simulink model "SoftStop_Standalone"  (R2022b)
settings: Solver=VariableStepAuto  StartTime=0.0  StopTime=10.0  RelTol=1e-3
undefined symbols (not defined in the file): AntiJerk_rear, iStop_Axle, iStop_ComfStop_Axis_SpeedAct_HA, iStop_ComfStop_Axis_SpeedActVA, iStop_ComfStop_TrqMinCont_HA, iStop_ComfStop_TrqMinCont_VA, iStop_HillComp_Axis_Steigung1, iStop_HillComp_Axis_Steigung2, iStop_HillComp_CompTrqFacHA, iStop_HillComp_CompTrqFacVA, iStop_HillComp_HillCompTrq, iStop_HillComp_HillEntrySpd, iStop_HillComp_HillExitPrs, iStop_HillComp_HillTrqLim_Dec_NegGrd, iStop_HillComp_HillTrqLim_Dec_PosGrd, iStop_HillComp_HillTrqLim_Inc_NegGrd, iStop_HillComp_HillTrqLim_Inc_PosGrd, iStop_Misc_SpeedLowr_Drive_Dir_HA, iStop_Misc_SpeedLowr_Drive_Dir_VA, iStop_Misc_SpeedUppr_Drive_Dir_HA, iStop_Misc_SpeedUppr_Drive_Dir_VA, iStop_PosCtrl_Activate_var_gain_HA, iStop_PosCtrl_Activate_var_gain_VA, iStop_PosCtrl_Actv_SpeedLowr_HA, iStop_PosCtrl_Actv_SpeedLowr_VA, iStop_PosCtrl_Actv_SpeedUppr_HA, iStop_PosCtrl_Actv_SpeedUppr_VA, iStop_PosCtrl_Axis_BrakeTorque_HA, iStop_PosCtrl_Axis_BrakeTorque_VA, iStop_PosCtrl_Axis_Delta_Speed_HA_Line, iStop_PosCtrl_Axis_Delta_Speed_HA_Map, iStop_PosCtrl_Axis_Delta_Speed_VA_Line, iStop_PosCtrl_Axis_Delta_Speed_VA_Map, iStop_PosCtrl_Axis_SpeedAct_VA, iStop_PosCtrl_Axis_SpeedActRear, iStop_PosCtrl_Axis_SpeedFilt_HA, iStop_PosCtrl_Axis_SpeedFilt_VA, iStop_PosCtrl_Gain_Line_HA, iStop_PosCtrl_Gain_Line_VA, iStop_PosCtrl_Gain_Map_HA, iStop_PosCtrl_Gain_Map_VA, iStop_PosCtrl_Hp_Filt_HA, iStop_PosCtrl_Hp_Filt_VA, iStop_PosCtrl_TrqOutput_PT1_HA, iStop_PosCtrl_TrqOutput_PT1_VA, iStop_SpeedLowrLim_Global_Actv, iStop_SpeedUpprLim_Global_Deactv, iStop_Standstill_Activate_hp_speed_filt_HA, iStop_Standstill_Activate_hp_speed_filt_VA, iStop_Standstill_Axis_PedalTravel, iStop_Standstill_Axis_SpeedAct_HA, iStop_Standstill_Axis_SpeedAct_VA, iStop_Standstill_delayHA, iStop_Standstill_delayVA, iStop_Standstill_Hp_Filt_HA, iStop_Standstill_Hp_Filt_VA, iStop_Standstill_MaxSpeedHA, iStop_Standstill_MaxSpeedVA, iStop_Standstill_MinSpeedHA, iStop_Standstill_MinSpeedVA ... (+2)
libraries: simulink x7, simulink_extras x6
settings Model: Creator=Z0186328  LastModifiedBy=Z0186328

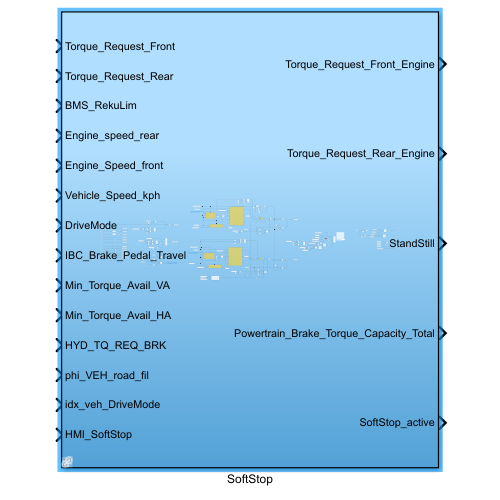
[thumbnail: Simulink's stored preview of the top-level diagram]
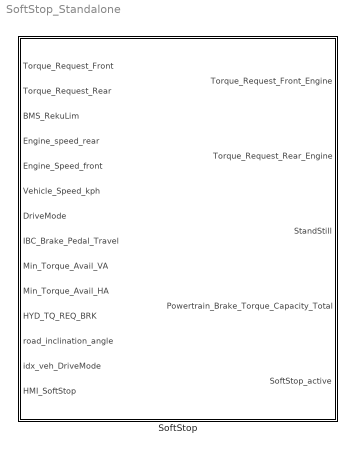
== system SoftStop_Standalone ==
  SoftStop : Subsystem  AncestorBlock=AntiJerk_rear/AntiJerk_rear

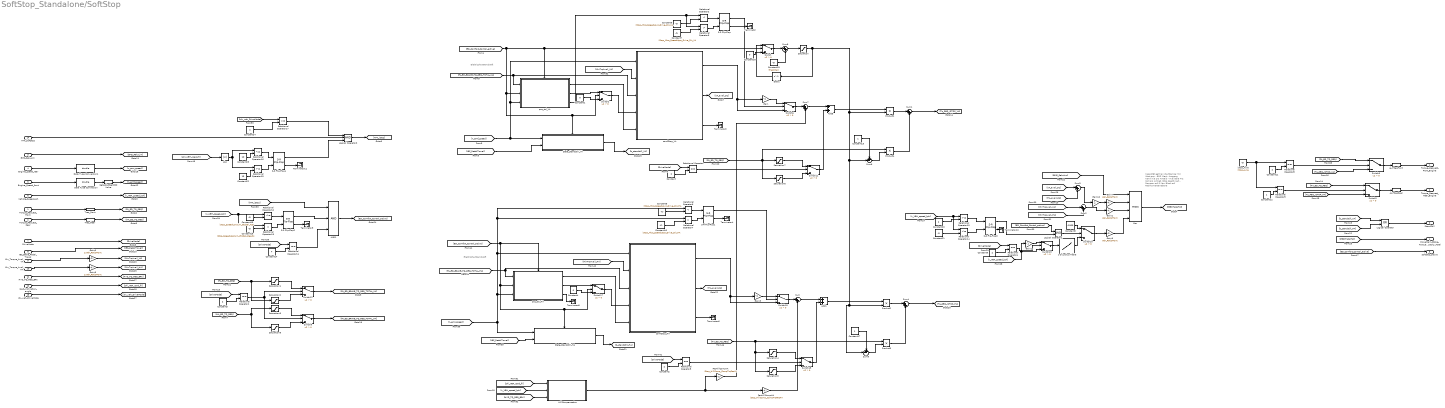
== system SoftStop_Standalone/SoftStop ==
  note: Elektrische Bremskraft
  note: Elektrische Bremskraft
  note: Kapazität geht an die Bremse:
      | Min Wert aus:
      | - BMS Wert
      | - Ausgang Kennlinie pro Antreib
      | - Available Trq CAN pro Antrieb
      |
      | IStop deaktiviert
      | - Rampen auf 0
      |
      | Max Block auf Radmomentenebene
  Torque_Request_Front : Inport
  Torque_Request_Rear : Inport  Port=2
  BMS_RekuLim : Inport  Port=3
  Engine_speed_rear : Inport  Port=4
  Engine_Speed_front : Inport  Port=5
  Vehicle_Speed_kph : Inport  Port=6
  DriveMode : Inport  Port=7
  IBC_Brake_Pedal_Travel : Inport  Port=8
  Min_Torque_Avail_VA : Inport  Port=9
  Min_Torque_Avail_HA : Inport  Port=10
  HYD_TQ_REQ_BRK : Inport  Port=11
  road_inclination_angle : Inport  Port=12
  idx_veh_DriveMode : Inport  Port=13
  HMI_SoftStop : Inport  Port=14
  1-D Lookup Table : Lookup_n-D  NumberOfTableDimensions=1  BreakpointsForDimension1=[0 8 12 15 20]  Table=[0 0 -250 -500 -1000]  ExtrapMethod=Clip  InternalRulePriority=Speed  RndMeth=Simplest
  AJ_TReqFront : SignalConversion  OverrideOpt=off
  AJ_TReqRear : SignalConversion  OverrideOpt=off
  AND1 : Logic  Inputs=3  AllPortsSameDT=off  OutDataTypeStr=boolean
  Abs : Abs  SaturateOnIntegerOverflow=off
  Add1 : Sum
  Add5 : Sum
  Constant{,2..3,9,11,20,24} (7 alike) : Constant  Value=2
  Constant1 : Constant  Value=0
  Constant10 : Constant  Value=iStop_Misc_SpeedUppr_Drive_Dir_HA
  Constant12 : Constant
  Constant13 : Constant
  Constant14 : Constant  Value=4
  Constant15 : Constant  Value=iStop_SpeedLowrLim_Global_Actv
  Constant16 : Constant  Value=iStop_SpeedUpprLim_Global_Deactv
  Constant17 : Constant
  Constant18 : Constant  Value=0
  Constant19 : Constant  Value=tTaskMain
  Constant21 : Constant  Value=-3
  Constant22 : Constant  Value=13
  Constant23 : Constant  Value=10
  Constant4 : Constant  Value=0
  Constant5 : Constant  Value=iStop_Misc_SpeedLowr_Drive_Dir_HA
  Constant6 : Constant  Value=iStop_Misc_SpeedLowr_Drive_Dir_VA
  Constant7 : Constant  Value=iStop_Misc_SpeedUppr_Drive_Dir_VA
  Constant8 : Constant  Value=-1000
  Data Type Conversion : DataTypeConversion  OutDataTypeStr=double  SaturateOnIntegerOverflow=off  RndMeth=Floor
  Data Type Conversion1 : DataTypeConversion  OutDataTypeStr=double  SaturateOnIntegerOverflow=off  RndMeth=Floor
  Delay : Delay  DelayLength=1  InitialCondition=0
  FacHillCompHA : Gain  Gain=iStop_HillComp_CompTrqFacHA
  FacHillCompVA : Gain  Gain=iStop_HillComp_CompTrqFacVA
  Gain : Gain  Gain=-1
  Gain1 : Gain  Gain=-1
  Gain10 : Gain  Gain=2
  Gain2 : Gain  Gain=Veh_RatioFront
  Gain3 : Gain  Gain=-1
  Gain6 : Gain  Gain=1/Veh_RatioFront
  Gain7 : Gain  Gain=Veh_RatioFront
  Gain8 : Gain  Gain=1/Veh_RatioFront
  Gain9 : Gain  Gain=Veh_RatioFront
  HillCompensation : Subsystem
  IsgSpdActSgn800 Value : SignalConversion  OverrideOpt=off
  Logical Operator : Logic  Operator=OR  AllPortsSameDT=off  OutDataTypeStr=boolean
  Logical Operator1 : Logic  AllPortsSameDT=off  OutDataTypeStr=boolean
  Logical Operator2 : Logic  Inputs=3  AllPortsSameDT=off  OutDataTypeStr=boolean
  Max : MinMax  Function=max  Inputs=4
  Product{1..4} (4 alike) : Product
  Relational Operator{,1,4..5,8..9,11} (7 alike) : RelationalOperator  Operator===  OutDataTypeStr=boolean  RndMeth=Simplest  InputSameDT=off
  Relational Operator10 : RelationalOperator  OutDataTypeStr=boolean  RndMeth=Simplest  InputSameDT=off
  Relational Operator{12,14,16..17} (4 alike) : RelationalOperator  Operator=<=  OutDataTypeStr=boolean  RndMeth=Simplest  InputSameDT=off
  Relational Operator13 : RelationalOperator  Operator=>  OutDataTypeStr=boolean  RndMeth=Simplest  InputSameDT=off
  Relational Operator15 : RelationalOperator  OutDataTypeStr=boolean  RndMeth=Simplest  InputSameDT=off
  Relational Operator2 : RelationalOperator  Operator=<  OutDataTypeStr=boolean  RndMeth=Simplest  InputSameDT=off
  Relational Operator3 : RelationalOperator  Operator=>  OutDataTypeStr=boolean  RndMeth=Simplest  InputSameDT=off
  Relational Operator6 : RelationalOperator  Operator=<  OutDataTypeStr=boolean  RndMeth=Simplest  InputSameDT=off
  Relational Operator7 : RelationalOperator  Operator=>  OutDataTypeStr=boolean  RndMeth=Simplest  InputSameDT=off
  S-R Flip-Flop{,1..4} (5 alike) : simulink_extras/Flip Flops/S-R Flip-Flop  initial_condition=0
  Saturation : Saturate  UpperLimit=1  LowerLimit=0
  Saturation{1,3,5..6} (4 alike) : Saturate  UpperLimit=inf  LowerLimit=0
  Saturation{2,4,7..8} (4 alike) : Saturate  UpperLimit=0  LowerLimit=-inf
  State_Standstill_HA : Subsystem
  State_Standstill_VA : Subsystem
  Sum{,1..4,7..8} (7 alike) : Sum  Inputs=|++
  Sum5 : Sum  Inputs=+-|
  Sum6 : Sum  Inputs=+-|
  Switch{,2..3,5..6,9..13,15,17..18} (13 alike) : Switch  Criteria=u2 > Threshold  SaturateOnIntegerOverflow=off  InputSameDT=off
  Terminator{,2,4,6,8..11} (8 alike) : Terminator
  Treq_Front : SignalConversion  OverrideOpt=off
  Treq_Rear : SignalConversion  OverrideOpt=off
  comfStop_HA : Subsystem
  comfStop_VA : Subsystem
  iStop_Axle : Constant  Value=iStop_Axle
  pos_ctrl_HA : Subsystem
  pos_ctrl_VA : Subsystem
  Torque_Request_Front_Engine : Outport
  Torque_Request_Rear_Engine : Outport  Port=2
  StandStill : Outport  Port=3
  Powertrain_Brake_Torque_Capacity_Total : Outport  Port=4
  SoftStop_active : Outport  Port=5
  wires:
  [ED_Comfort_Control_active] -> State_Standstill_HA/Enable, Switch17/2, pos_ctrl_HA/2(pos_ctrl_active), pos_ctrl_HA/Enable
  [ED_Comfort_Control_active] -> pos_ctrl_VA/Enable, Switch/2, Switch2/2, State_Standstill_VA/Enable, pos_ctrl_VA/2(pos_ctrl_active)
  Gain9/1 -> Max/4
  Gain7/1 -> Max/2
  Gain2/1 -> Max/3
  AJ_TReqRear/1 -> Torque_Request_Rear_Engine/1  "TReqRear"
  AJ_TReqFront/1 -> Torque_Request_Front_Engine/1  "TReqFront"
  Engine_Speed_front/1 -> Data Type Conversion/1
  Torque_Request_Rear/1 -> Treq_Rear/1
  Torque_Request_Front/1 -> Treq_Front/1
  Vehicle_Speed_kph/1 -> [v_VEH_speed_kph]
  IsgSpdActSgn800 Value/1 -> [n_emf_speed]
  Engine_speed_rear/1 -> Data Type Conversion1/1
  Saturation2/1 -> Switch12/3
  [DriveMode] -> Relational Operator1/1
  [FA_ED_TQ_REQ] -> Saturation1/1, Saturation2/1
  Saturation1/1 -> Switch12/1
  Saturation5/1 -> Switch9/1
  Saturation8/1 -> Switch9/3
  [HA_ED_TQ_REQ] -> Saturation5/1, Saturation8/1
  Relational Operator1/1 -> Switch12/2, Switch9/2
  Constant3/1 -> Relational Operator1/2
  Switch12/1 -> [FA_ED_BRAKE_TQ_REQ_TOTAL_VA]
  Switch9/1 -> [FA_ED_BRAKE_TQ_REQ_TOTAL_HA]
  [MinTrqAvail_HA] -> comfStop_HA/2(Tq_Avail_Min_HA)
  Relational Operator/1 -> Switch11/2
  Switch11/1 -> Add5/2
  Relational Operator3/1 -> S-R Flip-Flop/2
  [FA_ED_BRAKE_TQ_REQ_TOTAL_VA] -> comfStop_VA/3(ED_Brake_Tq_Req_VA_Total), pos_ctrl_VA/1(brake_torque_total)
  [DriveMode] -> Relational Operator/1
  S-R Flip-Flop/1 -> Switch6/2
  comfStop_VA/3(ED_Brake_Tq_VA_100%) -> Terminator2/1
  Constant2/1 -> Relational Operator5/2
  [DriveMode] -> Relational Operator5/1
  Constant/1 -> Relational Operator/2
  Constant6/1 -> Relational Operator2/2
  Constant7/1 -> Relational Operator3/2
  pos_ctrl_VA/3(speed_filt) -> Relational Operator2/1, Relational Operator3/1
  Relational Operator2/1 -> S-R Flip-Flop/1
  S-R Flip-Flop1/2 -> Terminator4/1
  Switch15/1 -> Add1/2
  Constant10/1 -> Relational Operator7/2
  Gain3/1 -> Switch18/1
  [n_emr_speed] -> comfStop_HA/1(Speed_Act_HA), Relational Operator7/1, Relational Operator6/1, pos_ctrl_HA/3(speed_act_HA), State_Standstill_HA/1(speed_act_HA)  "speed_act_HA"
  Relational Operator6/1 -> S-R Flip-Flop1/1
  comfStop_HA/2(HA_avail_trq) -> [HA_avail_trq]
  pos_ctrl_HA/2(position_control_trq_output_HA) -> Switch17/1
  Constant5/1 -> Relational Operator6/2
  State_Standstill_HA/1(stop_signal_after_integrator) -> [b_standstill_HA]  "stop_signal_active"
  [FA_ED_BRAKE_TQ_REQ_TOTAL_HA] -> comfStop_HA/3(ED_Brake_Tq_Req_HA_Total), pos_ctrl_HA/1(brake_torque_total)
  S-R Flip-Flop1/1 -> Switch18/2
  comfStop_HA/1(Brake_Tq_Req_HA_EDrive_Adjusted) -> Switch18/3, Gain3/1
  Saturation3/1 -> Switch15/3
  [n_emf_speed] -> State_Standstill_VA/1(speed_act_VA), pos_ctrl_VA/3(speed_act_VA), comfStop_VA/1(Speed_Act_VA)  "speed_act_VA"
  Constant4/1 -> Switch17/3
  comfStop_HA/3(ED_Brake_Tq_HA_100%) -> Terminator6/1
  [MinTrqAvail_VA] -> comfStop_VA/2(Tq_Avail_Min_VA)
  S-R Flip-Flop/2 -> Terminator/1
  Sum/1 -> Add1/1
  Gain/1 -> Switch6/1
  Saturation6/1 -> Switch11/3
  Saturation7/1 -> Switch11/1
  pos_ctrl_VA/2(position_control_trq_output_VA) -> Switch2/1
  Switch17/1 -> comfStop_HA/4(Pos_CRTL_TRQ_HA)
  Saturation4/1 -> Switch15/1
  Constant1/1 -> Switch2/3
  pos_ctrl_VA/1(pos_control_active_flag_VA) -> comfStop_VA/5(POS_CTRL_ACTIVE_VA)
  [FA_ED_TQ_REQ] -> Product4/1, Saturation6/1, Saturation7/1
  Relational Operator5/1 -> Switch15/2
  Sum7/1 -> Add5/1
  [IBC_PedalTravel] -> State_Standstill_VA/2(PedalTravel)
  Relational Operator7/1 -> S-R Flip-Flop1/2
  comfStop_VA/2(VA_avail_trq) -> [VA_avail_trq]
  pos_ctrl_HA/1(pos_control_active_flag_HA) -> comfStop_HA/5(POS_CTRL_ACTIVE_HA)
  Switch2/1 -> comfStop_VA/4(Pos_CRTL_TRQ_VA)
  comfStop_VA/1(Brake_Tq_Req_VA_EDrive_Adjusted) -> Gain/1, Switch6/3
  [IBC_PedalTravel] -> State_Standstill_HA/2(PedalTravel)
  pos_ctrl_HA/3(speed_filt) -> Terminator8/1
  State_Standstill_VA/1(stop_signal_after_integrator) -> [b_standstill_VA]  "stop_signal_active"
  1-D Lookup Table/1 -> Switch10/3
  Switch13/1 -> 1-D Lookup Table/1
  Gain1/1 -> Switch13/1
  [MinTrqAvail_VA] -> Sum2/1
  [BMS_RekuLim] -> Max/1
  Sum3/1 -> Gain10/1
  Logical Operator1/1 -> Switch10/2
  Relational Operator4/1 -> Switch13/2
  [v_VEH_speed_kph] -> Gain1/1, Switch13/3
  Constant8/1 -> Switch10/1
  Sum2/1 -> Gain2/1
  Switch10/1 -> Gain9/1
  [HA_avail_trq] -> Sum3/2
  [DriveMode] -> Relational Operator4/1
  Max/1 -> [PtBrkTqCpTot]
  Constant9/1 -> Relational Operator4/2
  [MinTrqAvail_HA] -> Sum2/2
  [VA_avail_trq] -> Sum3/1
  [b_standstill_HA] -> Logical Operator/2  "b_StandStill"
  [PtBrkTqCpTot] -> Powertrain_Brake_Torque_Capacity_Total/1  "PtBrkTqCpTot"
  [b_standstill_VA] -> Logical Operator/1  "b_StandStill"
  Switch3/1 -> AJ_TReqRear/1
  [FA_ED_TQ_REQ] -> Switch5/1
  [HA_ED_TQ_REQ] -> Switch3/1
  Switch5/1 -> AJ_TReqFront/1
  Relational Operator8/1 -> Switch5/2
  Constant12/1 -> Relational Operator9/2
  [Tq_REQ_ISTOP_HA] -> Switch3/3
  [Tq_REQ_ISTOP_VA] -> Switch5/3
  Constant11/1 -> Relational Operator8/2
  Relational Operator9/1 -> Switch3/2
  iStop_Axle/1 -> Relational Operator9/1, Relational Operator8/1
  Treq_Front/1 -> [FA_ED_TQ_REQ]  "AJ_TReqFront"
  Treq_Rear/1 -> [HA_ED_TQ_REQ]
  IBC_Brake_Pedal_Travel/1 -> [IBC_PedalTravel]
  Logical Operator2/1 -> [HMI_iStop]
  DriveMode/1 -> [DriveMode]
  BMS_RekuLim/1 -> [BMS_RekuLim]
  Min_Torque_Avail_VA/1 -> Gain6/1
  Min_Torque_Avail_HA/1 -> Gain8/1
  Gain6/1 -> [MinTrqAvail_VA]
  Gain8/1 -> [MinTrqAvail_HA]
  Logical Operator/1 -> StandStill/1  "b_StandStill"
  HYD_TQ_REQ_BRK/1 -> [HYD_TQ_REQ_BRK]  "IBC_SRBM_IST"
  Data Type Conversion1/1 -> [n_emr_speed]
  Data Type Conversion/1 -> IsgSpdActSgn800 Value/1
  Relational Operator11/1 -> AND1/3
  Constant15/1 -> Relational Operator12/2
  [v_VEH_speed_kph] -> Relational Operator12/1, Relational Operator13/1
  Constant19/1 -> Sum8/2
  Relational Operator13/1 -> S-R Flip-Flop2/2
  Switch/1 -> Sum8/1
  S-R Flip-Flop2/1 -> AND1/2
  Constant18/1 -> Switch/3
  [HMI_iStop] -> AND1/1
  Delay/1 -> Switch/1
  Sum8/1 -> Saturation/1
  AND1/1 -> [ED_Comfort_Control_active]
  [DriveMode] -> Relational Operator11/1
  Relational Operator12/1 -> S-R Flip-Flop2/1
  Constant16/1 -> Relational Operator13/2
  Constant14/1 -> Relational Operator11/2
  S-R Flip-Flop2/2 -> Terminator9/1
  Sum4/1 -> [Tq_REQ_ISTOP_HA]
  Add1/1 -> Product2/1
  Product2/1 -> Sum4/1
  Product3/1 -> Sum4/2
  [HA_ED_TQ_REQ] -> Saturation3/1, Saturation4/1, Product3/1
  Constant17/1 -> Sum5/1
  Sum5/1 -> Product3/2
  Sum6/1 -> Product4/2
  Saturation/1 -> Product1/2, Sum5/2, Product2/2, Sum6/2, Delay/1  "ED_Comfort_Control_active_interpol"
  Constant13/1 -> Sum6/1
  Product4/1 -> Sum1/2
  Product1/1 -> Sum1/1
  Add5/1 -> Product1/1
  Sum1/1 -> [Tq_REQ_ISTOP_VA]
  Switch18/1 -> Sum/1
  [v_VEH_speed_kph] -> HillCompensation/2(Speed)
  [HYD_TQ_REQ_BRK] -> HillCompensation/3(BrakePressure)
  [phi_VEH_road_fil] -> HillCompensation/1(Steigung)
  HillCompensation/1(trq_hillcomp) -> FacHillCompHA/1, FacHillCompVA/1
  road_inclination_angle/1 -> [phi_VEH_road_fil]
  [v_VEH_speed_kph] -> Relational Operator10/1, Relational Operator14/1
  S-R Flip-Flop3/2 -> Terminator10/1
  Constant21/1 -> Relational Operator14/2
  Relational Operator10/1 -> S-R Flip-Flop3/1
  [ED_Comfort_Control_active] -> Logical Operator1/1
  Relational Operator14/1 -> S-R Flip-Flop3/2
  S-R Flip-Flop3/1 -> Logical Operator1/2
  Constant20/1 -> Relational Operator10/2
  FacHillCompHA/1 -> Sum/2
  Switch6/1 -> Sum7/1
  FacHillCompVA/1 -> Sum7/2
  [ED_Comfort_Control_active] -> SoftStop_active/1  "ED_Comfort_Control_active"
  S-R Flip-Flop4/1 -> Logical Operator2/3
  S-R Flip-Flop4/2 -> Terminator11/1
  [phi_VEH_road_fil] -> Abs/1
  Relational Operator15/1 -> S-R Flip-Flop4/2
  Constant22/1 -> Relational Operator15/2
  Abs/1 -> Relational Operator16/1, Relational Operator15/1
  Relational Operator16/1 -> S-R Flip-Flop4/1
  Constant23/1 -> Relational Operator16/2
  Constant24/1 -> Relational Operator17/2
  Relational Operator17/1 -> Logical Operator2/1
  idx_veh_DriveMode/1 -> [idx_veh_DriveMode]
  [idx_veh_DriveMode] -> Relational Operator17/1
  Gain10/1 -> Gain7/1
  HMI_SoftStop/1 -> Logical Operator2/2

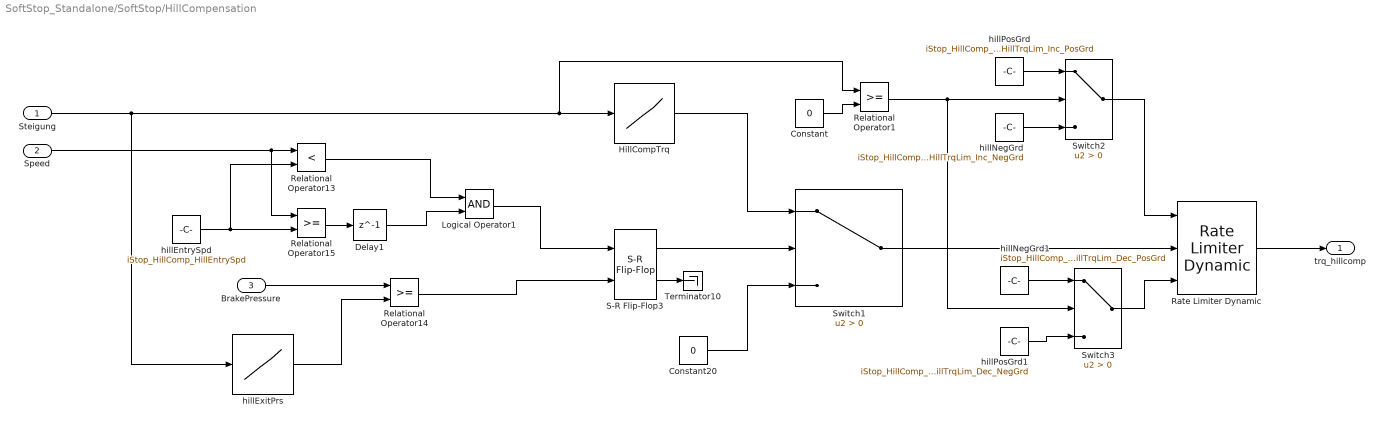
== system SoftStop_Standalone/SoftStop/HillCompensation ==
  Steigung : Inport
  Speed : Inport  Port=2
  BrakePressure : Inport  Port=3
  Constant : Constant  Value=0
  Constant20 : Constant  Value=0
  Delay1 : Delay  DelayLength=1  InitialCondition=0
  HillCompTrq : Lookup_n-D  NumberOfTableDimensions=1  BreakpointsForDimension1=iStop_HillComp_Axis_Steigung2  Table=iStop_HillComp_HillCompTrq  ExtrapMethod=Clip  UseLastTableValue=on  InternalRulePriority=Speed  RndMeth=Simplest
  Logical Operator1 : Logic  AllPortsSameDT=off  OutDataTypeStr=boolean
  Rate Limiter Dynamic : simulink/Discontinuities/Rate Limiter Dynamic
  Relational Operator1 : RelationalOperator  OutDataTypeStr=boolean  RndMeth=Simplest  InputSameDT=off
  Relational Operator13 : RelationalOperator  Operator=<  OutDataTypeStr=boolean  RndMeth=Simplest  InputSameDT=off
  Relational Operator14 : RelationalOperator  OutDataTypeStr=boolean  RndMeth=Simplest  InputSameDT=off
  Relational Operator15 : RelationalOperator  OutDataTypeStr=boolean  RndMeth=Simplest  InputSameDT=off
  S-R Flip-Flop3 : simulink_extras/Flip Flops/S-R Flip-Flop  initial_condition=0
  Switch1 : Switch  Criteria=u2 > Threshold  SaturateOnIntegerOverflow=off  InputSameDT=off
  Switch2 : Switch  Criteria=u2 > Threshold  SaturateOnIntegerOverflow=off  InputSameDT=off
  Switch3 : Switch  Criteria=u2 > Threshold  SaturateOnIntegerOverflow=off  InputSameDT=off
  Terminator10 : Terminator
  hillEntrySpd : Constant  Value=iStop_HillComp_HillEntrySpd
  hillExitPrs : Lookup_n-D  NumberOfTableDimensions=1  BreakpointsForDimension1=iStop_HillComp_Axis_Steigung1  Table=iStop_HillComp_HillExitPrs  ExtrapMethod=Clip  UseLastTableValue=on  InternalRulePriority=Speed  RndMeth=Simplest
  hillNegGrd : Constant  Value=iStop_HillComp_HillTrqLim_Inc_NegGrd
  hillNegGrd1 : Constant  Value=iStop_HillComp_HillTrqLim_Dec_PosGrd
  hillPosGrd : Constant  Value=iStop_HillComp_HillTrqLim_Inc_PosGrd
  hillPosGrd1 : Constant  Value=iStop_HillComp_HillTrqLim_Dec_NegGrd
  trq_hillcomp : Outport
  wires:
  hillPosGrd1/1 -> Switch3/3
  hillNegGrd1/1 -> Switch3/1
  Constant/1 -> Relational Operator1/2
  Relational Operator1/1 -> Switch2/2, Switch3/2
  Switch3/1 -> Rate Limiter Dynamic/3
  hillNegGrd/1 -> Switch2/3
  Switch2/1 -> Rate Limiter Dynamic/1
  hillPosGrd/1 -> Switch2/1
  BrakePressure/1 -> Relational Operator14/1
  Switch1/1 -> Rate Limiter Dynamic/2
  Logical Operator1/1 -> S-R Flip-Flop3/1
  hillExitPrs/1 -> Relational Operator14/2
  Rate Limiter Dynamic/1 -> trq_hillcomp/1
  Delay1/1 -> Logical Operator1/2
  Relational Operator14/1 -> S-R Flip-Flop3/2
  Steigung/1 -> HillCompTrq/1, Relational Operator1/1, hillExitPrs/1
  HillCompTrq/1 -> Switch1/1
  Constant20/1 -> Switch1/3
  Relational Operator15/1 -> Delay1/1
  S-R Flip-Flop3/1 -> Switch1/2
  Speed/1 -> Relational Operator13/1, Relational Operator15/1
  Relational Operator13/1 -> Logical Operator1/1
  S-R Flip-Flop3/2 -> Terminator10/1
  hillEntrySpd/1 -> Relational Operator15/2, Relational Operator13/2

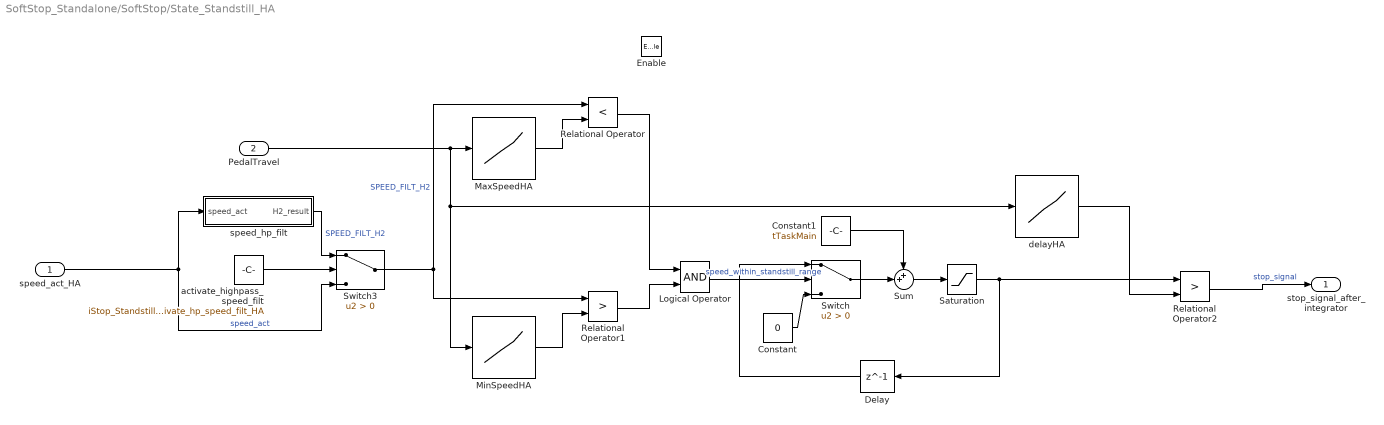
== system SoftStop_Standalone/SoftStop/State_Standstill_HA ==
  speed_act_HA : Inport
  PedalTravel : Inport  Port=2
  Enable : EnablePort  StatesWhenEnabling=reset
  Constant : Constant  Value=0
  Constant1 : Constant  Value=tTaskMain
  Delay : Delay  DelayLength=1  InitialCondition=0
  Logical Operator : Logic  AllPortsSameDT=off  OutDataTypeStr=boolean
  MaxSpeedHA : Lookup_n-D  NumberOfTableDimensions=1  BreakpointsForDimension1=iStop_Standstill_Axis_PedalTravel  Table=iStop_Standstill_MaxSpeedHA  ExtrapMethod=Clip  UseLastTableValue=on  InternalRulePriority=Speed  RndMeth=Simplest
  MinSpeedHA : Lookup_n-D  NumberOfTableDimensions=1  BreakpointsForDimension1=iStop_Standstill_Axis_PedalTravel  Table=iStop_Standstill_MinSpeedHA  ExtrapMethod=Clip  UseLastTableValue=on  InternalRulePriority=Speed  RndMeth=Simplest
  Relational Operator : RelationalOperator  Operator=<  OutDataTypeStr=boolean  RndMeth=Simplest  InputSameDT=off
  Relational Operator1 : RelationalOperator  Operator=>  OutDataTypeStr=boolean  RndMeth=Simplest  InputSameDT=off
  Relational Operator2 : RelationalOperator  Operator=>  OutDataTypeStr=boolean  RndMeth=Simplest  InputSameDT=off
  Saturation : Saturate  UpperLimit=10  LowerLimit=0
  Sum : Sum  Inputs=++|
  Switch : Switch  Criteria=u2 > Threshold  SaturateOnIntegerOverflow=off  InputSameDT=off
  Switch3 : Switch  Criteria=u2 > Threshold  SaturateOnIntegerOverflow=off  InputSameDT=off
  activate_highpass_speed_filt : Constant  Value=iStop_Standstill_Activate_hp_speed_filt_HA
  delayHA : Lookup_n-D  NumberOfTableDimensions=1  BreakpointsForDimension1=iStop_Standstill_Axis_PedalTravel  Table=iStop_Standstill_delayHA  ExtrapMethod=Clip  UseLastTableValue=on  InternalRulePriority=Speed  RndMeth=Simplest
  speed_hp_filt : Subsystem
  stop_signal_after_integrator : Outport
  wires:
  delayHA/1 -> Relational Operator2/2
  MinSpeedHA/1 -> Relational Operator1/2
  Relational Operator1/1 -> Logical Operator/2
  PedalTravel/1 -> MaxSpeedHA/1, delayHA/1, MinSpeedHA/1
  MaxSpeedHA/1 -> Relational Operator/2
  Relational Operator2/1 -> stop_signal_after_integrator/1  "stop_signal"
  Logical Operator/1 -> Switch/2  "speed_within_standstill_range"
  Relational Operator/1 -> Logical Operator/1
  speed_act_HA/1 -> Switch3/3, speed_hp_filt/1(speed_act)  "speed_act"
  speed_hp_filt/1(H2_result) -> Switch3/1  "SPEED_FILT_H2"
  activate_highpass_speed_filt/1 -> Switch3/2
  Switch3/1 -> Relational Operator/1, Relational Operator1/1  "SPEED_FILT_H2"
  Constant/1 -> Switch/3
  Delay/1 -> Switch/1
  Switch/1 -> Sum/2
  Sum/1 -> Saturation/1
  Constant1/1 -> Sum/1
  Saturation/1 -> Relational Operator2/1, Delay/1

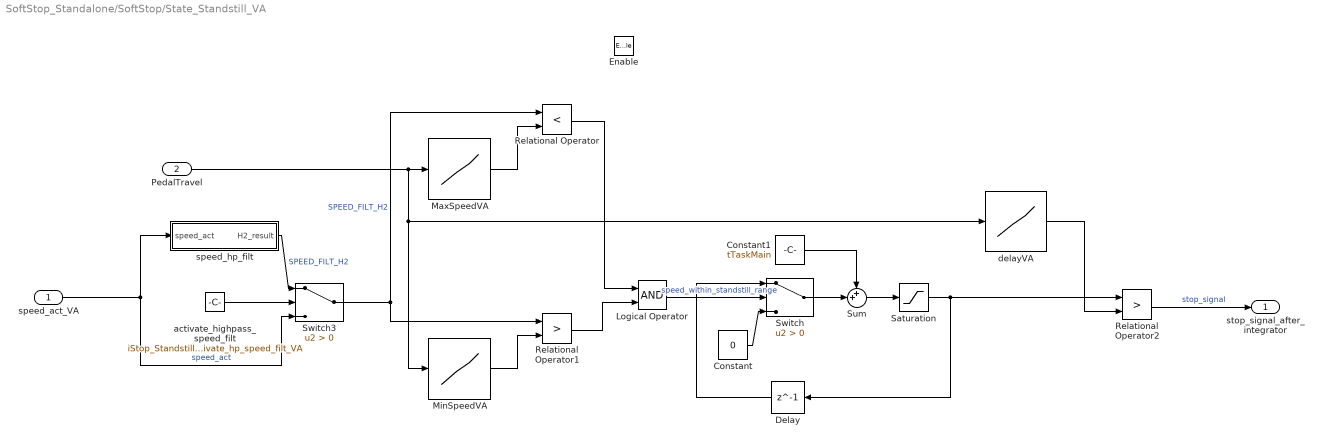
== system SoftStop_Standalone/SoftStop/State_Standstill_VA ==
  speed_act_VA : Inport
  PedalTravel : Inport  Port=2
  Enable : EnablePort  StatesWhenEnabling=reset
  Constant : Constant  Value=0
  Constant1 : Constant  Value=tTaskMain
  Delay : Delay  DelayLength=1  InitialCondition=0
  Logical Operator : Logic  AllPortsSameDT=off  OutDataTypeStr=boolean
  MaxSpeedVA : Lookup_n-D  NumberOfTableDimensions=1  BreakpointsForDimension1=iStop_Standstill_Axis_PedalTravel  Table=iStop_Standstill_MaxSpeedVA  ExtrapMethod=Clip  UseLastTableValue=on  InternalRulePriority=Speed  RndMeth=Simplest
  MinSpeedVA : Lookup_n-D  NumberOfTableDimensions=1  BreakpointsForDimension1=iStop_Standstill_Axis_PedalTravel  Table=iStop_Standstill_MinSpeedVA  ExtrapMethod=Clip  UseLastTableValue=on  InternalRulePriority=Speed  RndMeth=Simplest
  Relational Operator : RelationalOperator  Operator=<  OutDataTypeStr=boolean  RndMeth=Simplest  InputSameDT=off
  Relational Operator1 : RelationalOperator  Operator=>  OutDataTypeStr=boolean  RndMeth=Simplest  InputSameDT=off
  Relational Operator2 : RelationalOperator  Operator=>  OutDataTypeStr=boolean  RndMeth=Simplest  InputSameDT=off
  Saturation : Saturate  UpperLimit=10  LowerLimit=0
  Sum : Sum  Inputs=++|
  Switch : Switch  Criteria=u2 > Threshold  SaturateOnIntegerOverflow=off  InputSameDT=off
  Switch3 : Switch  Criteria=u2 > Threshold  SaturateOnIntegerOverflow=off  InputSameDT=off
  activate_highpass_speed_filt : Constant  Value=iStop_Standstill_Activate_hp_speed_filt_VA
  delayVA : Lookup_n-D  NumberOfTableDimensions=1  BreakpointsForDimension1=iStop_Standstill_Axis_PedalTravel  Table=iStop_Standstill_delayVA  ExtrapMethod=Clip  UseLastTableValue=on  InternalRulePriority=Speed  RndMeth=Simplest
  speed_hp_filt : Subsystem
  stop_signal_after_integrator : Outport
  wires:
  Switch3/1 -> Relational Operator1/1, Relational Operator/1  "SPEED_FILT_H2"
  activate_highpass_speed_filt/1 -> Switch3/2
  speed_hp_filt/1(H2_result) -> Switch3/1  "SPEED_FILT_H2"
  speed_act_VA/1 -> Switch3/3, speed_hp_filt/1(speed_act)  "speed_act"
  Relational Operator/1 -> Logical Operator/1
  Relational Operator2/1 -> stop_signal_after_integrator/1  "stop_signal"
  MaxSpeedVA/1 -> Relational Operator/2
  PedalTravel/1 -> MinSpeedVA/1, delayVA/1, MaxSpeedVA/1
  Relational Operator1/1 -> Logical Operator/2
  MinSpeedVA/1 -> Relational Operator1/2
  delayVA/1 -> Relational Operator2/2
  Switch/1 -> Sum/2
  Constant/1 -> Switch/3
  Saturation/1 -> Relational Operator2/1, Delay/1
  Constant1/1 -> Sum/1
  Logical Operator/1 -> Switch/2  "speed_within_standstill_range"
  Sum/1 -> Saturation/1
  Delay/1 -> Switch/1

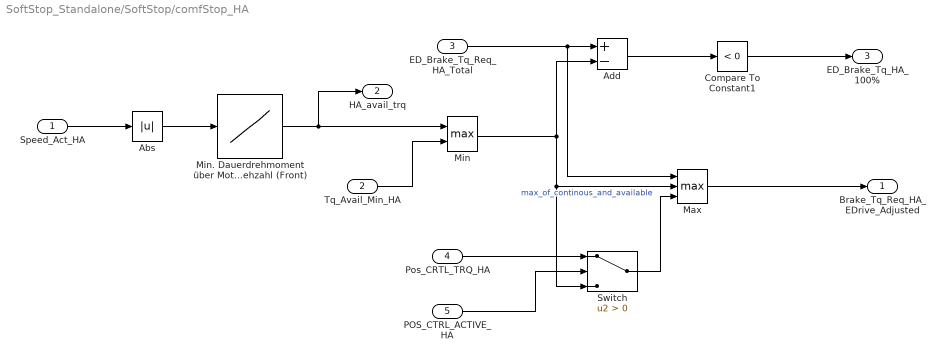
== system SoftStop_Standalone/SoftStop/comfStop_HA ==
  Speed_Act_HA : Inport
  Tq_Avail_Min_HA : Inport  Port=2
  ED_Brake_Tq_Req_HA_Total : Inport  Port=3
  Pos_CRTL_TRQ_HA : Inport  Port=4
  POS_CTRL_ACTIVE_HA : Inport  Port=5
  Abs : Abs  SaturateOnIntegerOverflow=off
  Add : Sum  Inputs=+-
  Compare To Constant1 : simulink/Logic and Bit Operations/Compare To Constant  relop=<  const=0  OutDataTypeStr=boolean
  Max : MinMax  Function=max  Inputs=3
  Min : MinMax  Function=max  Inputs=2
  Min. Dauerdrehmoment über Motordrehzahl (Front) : Lookup_n-D  NumberOfTableDimensions=1  BreakpointsForDimension1=iStop_ComfStop_Axis_SpeedAct_HA  Table=iStop_ComfStop_TrqMinCont_HA  ExtrapMethod=Clip  UseLastTableValue=on  InternalRulePriority=Speed  RndMeth=Simplest
  Switch : Switch  Criteria=u2 > Threshold  SaturateOnIntegerOverflow=off  InputSameDT=off
  Brake_Tq_Req_HA_EDrive_Adjusted : Outport
  HA_avail_trq : Outport  Port=2
  ED_Brake_Tq_HA_100% : Outport  Port=3
  wires:
  Add/1 -> Compare To Constant1/1
  Min. Dauerdrehmoment über Motordrehzahl (Front)/1 -> HA_avail_trq/1, Min/1
  ED_Brake_Tq_Req_HA_Total/1 -> Max/1, Add/1
  Tq_Avail_Min_HA/1 -> Min/2
  Min/1 -> Switch/3, Max/2, Add/2  "max_of_continous_and_available"
  Speed_Act_HA/1 -> Abs/1
  Max/1 -> Brake_Tq_Req_HA_EDrive_Adjusted/1
  POS_CTRL_ACTIVE_HA/1 -> Switch/2
  Pos_CRTL_TRQ_HA/1 -> Switch/1
  Switch/1 -> Max/3
  Compare To Constant1/1 -> ED_Brake_Tq_HA_100%/1
  Abs/1 -> Min. Dauerdrehmoment über Motordrehzahl (Front)/1

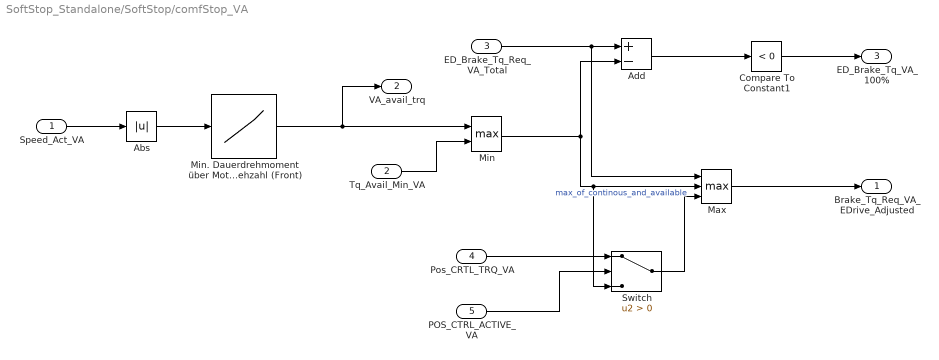
== system SoftStop_Standalone/SoftStop/comfStop_VA ==
  Speed_Act_VA : Inport
  Tq_Avail_Min_VA : Inport  Port=2
  ED_Brake_Tq_Req_VA_Total : Inport  Port=3
  Pos_CRTL_TRQ_VA : Inport  Port=4
  POS_CTRL_ACTIVE_VA : Inport  Port=5
  Abs : Abs  SaturateOnIntegerOverflow=off
  Add : Sum  Inputs=+-
  Compare To Constant1 : simulink/Logic and Bit Operations/Compare To Constant  relop=<  const=0  OutDataTypeStr=boolean
  Max : MinMax  Function=max  Inputs=3
  Min : MinMax  Function=max  Inputs=2
  Min. Dauerdrehmoment über Motordrehzahl (Front) : Lookup_n-D  NumberOfTableDimensions=1  BreakpointsForDimension1=iStop_ComfStop_Axis_SpeedActVA  Table=iStop_ComfStop_TrqMinCont_VA  ExtrapMethod=Clip  UseLastTableValue=on  InternalRulePriority=Speed  RndMeth=Simplest
  Switch : Switch  Criteria=u2 > Threshold  SaturateOnIntegerOverflow=off  InputSameDT=off
  Brake_Tq_Req_VA_EDrive_Adjusted : Outport
  VA_avail_trq : Outport  Port=2
  ED_Brake_Tq_VA_100% : Outport  Port=3
  wires:
  Add/1 -> Compare To Constant1/1
  Min. Dauerdrehmoment über Motordrehzahl (Front)/1 -> VA_avail_trq/1, Min/1
  ED_Brake_Tq_Req_VA_Total/1 -> Max/1, Add/1
  Tq_Avail_Min_VA/1 -> Min/2
  Min/1 -> Switch/3, Max/2, Add/2  "max_of_continous_and_available"
  Speed_Act_VA/1 -> Abs/1
  Max/1 -> Brake_Tq_Req_VA_EDrive_Adjusted/1
  POS_CTRL_ACTIVE_VA/1 -> Switch/2
  Pos_CRTL_TRQ_VA/1 -> Switch/1
  Switch/1 -> Max/3
  Compare To Constant1/1 -> ED_Brake_Tq_VA_100%/1
  Abs/1 -> Min. Dauerdrehmoment über Motordrehzahl (Front)/1

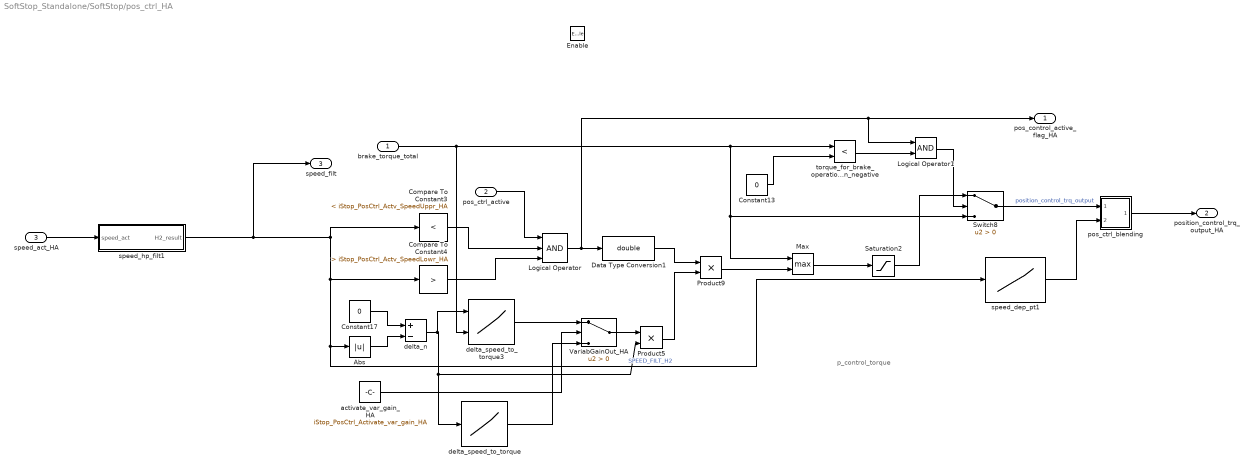
== system SoftStop_Standalone/SoftStop/pos_ctrl_HA ==
  note: p_control_torque
  brake_torque_total : Inport
  pos_ctrl_active : Inport  Port=2
  speed_act_HA : Inport  Port=3
  Enable : EnablePort  StatesWhenEnabling=reset
  Abs : Abs  SaturateOnIntegerOverflow=off
  Compare To Constant3 : simulink/Logic and Bit Operations/Compare To Constant  relop=<  const=iStop_PosCtrl_Actv_SpeedUppr_HA  OutDataTypeStr=boolean
  Compare To Constant4 : simulink/Logic and Bit Operations/Compare To Constant  relop=>  const=iStop_PosCtrl_Actv_SpeedLowr_HA  OutDataTypeStr=boolean
  Constant13 : Constant  Value=0
  Constant17 : Constant  Value=0
  Data Type Conversion1 : DataTypeConversion  OutDataTypeStr=double  SaturateOnIntegerOverflow=off  RndMeth=Floor
  Logical Operator : Logic  Inputs=3  AllPortsSameDT=off  OutDataTypeStr=boolean
  Logical Operator1 : Logic  AllPortsSameDT=off  OutDataTypeStr=boolean
  Max : MinMax  Function=max  Inputs=2
  Product5 : Product
  Product9 : Product
  Saturation2 : Saturate  UpperLimit=0  LowerLimit=-250
  Switch8 : Switch  Criteria=u2 > Threshold  SaturateOnIntegerOverflow=off  InputSameDT=off
  VariabGainOut_HA : Switch  Criteria=u2 > Threshold  SaturateOnIntegerOverflow=off  InputSameDT=off
  activate_var_gain_HA : Constant  Value=iStop_PosCtrl_Activate_var_gain_HA
  delta_n : Sum  Inputs=+-
  delta_speed_to_torque : Lookup_n-D  NumberOfTableDimensions=1  BreakpointsForDimension1=iStop_PosCtrl_Axis_Delta_Speed_HA_Line  Table=iStop_PosCtrl_Gain_Line_HA  ExtrapMethod=Clip  UseLastTableValue=on  InternalRulePriority=Speed  RndMeth=Simplest
  delta_speed_to_torque3 : Lookup_n-D  BreakpointsForDimension1=iStop_PosCtrl_Axis_Delta_Speed_HA_Map  BreakpointsForDimension2=iStop_PosCtrl_Axis_BrakeTorque_HA  Table=iStop_PosCtrl_Gain_Map_HA  ExtrapMethod=Clip  UseLastTableValue=on  InternalRulePriority=Speed  RndMeth=Simplest
      settings: InputPortMap=u0,u1
  pos_ctrl_blending : Subsystem
  speed_dep_pt1 : Lookup_n-D  NumberOfTableDimensions=1  BreakpointsForDimension1=iStop_PosCtrl_Axis_SpeedFilt_HA  Table=iStop_PosCtrl_TrqOutput_PT1_HA  ExtrapMethod=Clip  UseLastTableValue=on  InternalRulePriority=Speed  RndMeth=Simplest
  speed_hp_filt1 : Subsystem
  torque_for_brake_operation_sign_negative : RelationalOperator  Operator=<  OutDataTypeStr=boolean  RndMeth=Simplest  InputSameDT=off
  pos_control_active_flag_HA : Outport
  position_control_trq_output_HA : Outport  Port=2
  speed_filt : Outport  Port=3
  wires:
  speed_hp_filt1/1(H2_result) -> speed_filt/1, Compare To Constant3/1, Compare To Constant4/1, Abs/1, speed_dep_pt1/1  "SPEED_FILT_H2"
  speed_act_HA/1 -> speed_hp_filt1/1(speed_act)
  speed_dep_pt1/1 -> pos_ctrl_blending/2(In2)
  Compare To Constant4/1 -> Logical Operator/3
  Logical Operator/1 -> Data Type Conversion1/1, pos_control_active_flag_HA/1, Logical Operator1/1
  Switch8/1 -> pos_ctrl_blending/1(In1)  "position_control_trq_output"
  delta_speed_to_torque/1 -> VariabGainOut_HA/3
  Logical Operator1/1 -> Switch8/2
  Max/1 -> Saturation2/1
  Product9/1 -> Max/2
  torque_for_brake_operation_sign_negative/1 -> Logical Operator1/2
  Data Type Conversion1/1 -> Product9/1
  Product5/1 -> Product9/2
  pos_ctrl_active/1 -> Logical Operator/1
  Saturation2/1 -> Switch8/1
  Abs/1 -> delta_n/2
  Constant17/1 -> delta_n/1
  pos_ctrl_blending/1(Out1) -> position_control_trq_output_HA/1
  delta_n/1 -> delta_speed_to_torque3/1, delta_speed_to_torque/1, Product5/2
  Compare To Constant3/1 -> Logical Operator/2
  Constant13/1 -> torque_for_brake_operation_sign_negative/2
  activate_var_gain_HA/1 -> VariabGainOut_HA/2
  delta_speed_to_torque3/1 -> VariabGainOut_HA/1
  brake_torque_total/1 -> delta_speed_to_torque3/2, torque_for_brake_operation_sign_negative/1, Max/1, Switch8/3
  VariabGainOut_HA/1 -> Product5/1

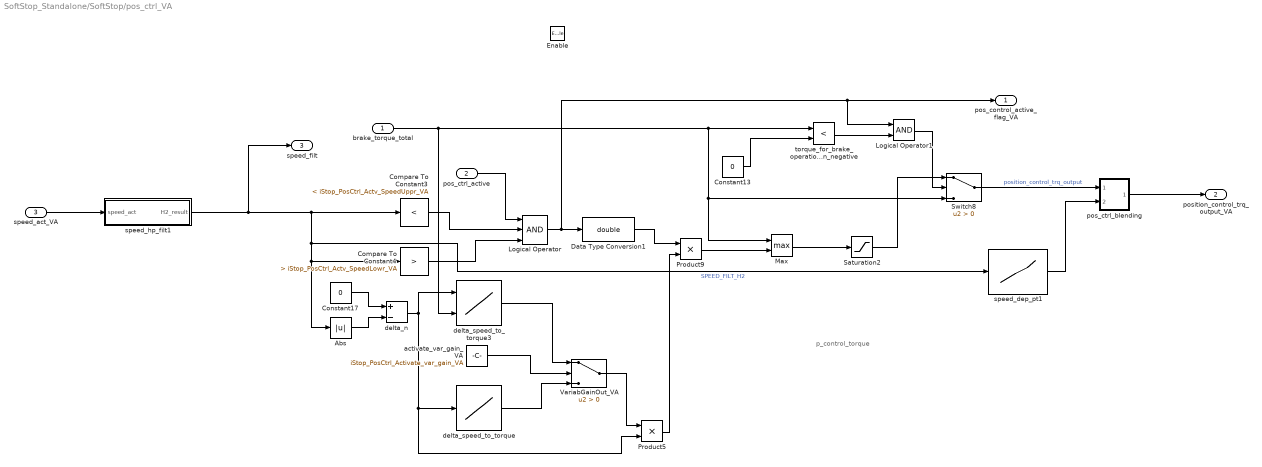
== system SoftStop_Standalone/SoftStop/pos_ctrl_VA ==
  note: p_control_torque
  brake_torque_total : Inport
  pos_ctrl_active : Inport  Port=2
  speed_act_VA : Inport  Port=3
  Enable : EnablePort  StatesWhenEnabling=reset
  Abs : Abs  SaturateOnIntegerOverflow=off
  Compare To Constant3 : simulink/Logic and Bit Operations/Compare To Constant  relop=<  const=iStop_PosCtrl_Actv_SpeedUppr_VA  OutDataTypeStr=boolean
  Compare To Constant4 : simulink/Logic and Bit Operations/Compare To Constant  relop=>  const=iStop_PosCtrl_Actv_SpeedLowr_VA  OutDataTypeStr=boolean
  Constant13 : Constant  Value=0
  Constant17 : Constant  Value=0
  Data Type Conversion1 : DataTypeConversion  OutDataTypeStr=double  SaturateOnIntegerOverflow=off  RndMeth=Floor
  Logical Operator : Logic  Inputs=3  AllPortsSameDT=off  OutDataTypeStr=boolean
  Logical Operator1 : Logic  AllPortsSameDT=off  OutDataTypeStr=boolean
  Max : MinMax  Function=max  Inputs=2
  Product5 : Product
  Product9 : Product
  Saturation2 : Saturate  UpperLimit=0  LowerLimit=-250
  Switch8 : Switch  Criteria=u2 > Threshold  SaturateOnIntegerOverflow=off  InputSameDT=off
  VariabGainOut_VA : Switch  Criteria=u2 > Threshold  SaturateOnIntegerOverflow=off  InputSameDT=off
  activate_var_gain_VA : Constant  Value=iStop_PosCtrl_Activate_var_gain_VA
  delta_n : Sum  Inputs=+-
  delta_speed_to_torque : Lookup_n-D  NumberOfTableDimensions=1  BreakpointsForDimension1=iStop_PosCtrl_Axis_Delta_Speed_VA_Line  Table=iStop_PosCtrl_Gain_Line_VA  ExtrapMethod=Clip  UseLastTableValue=on  InternalRulePriority=Speed  RndMeth=Simplest
  delta_speed_to_torque3 : Lookup_n-D  BreakpointsForDimension1=iStop_PosCtrl_Axis_Delta_Speed_VA_Map  BreakpointsForDimension2=iStop_PosCtrl_Axis_BrakeTorque_VA  Table=iStop_PosCtrl_Gain_Map_VA  ExtrapMethod=Clip  UseLastTableValue=on  InternalRulePriority=Speed  RndMeth=Simplest
      settings: InputPortMap=u0,u1
  pos_ctrl_blending : Subsystem
  speed_dep_pt1 : Lookup_n-D  NumberOfTableDimensions=1  BreakpointsForDimension1=iStop_PosCtrl_Axis_SpeedFilt_VA  Table=iStop_PosCtrl_TrqOutput_PT1_VA  ExtrapMethod=Clip  UseLastTableValue=on  InternalRulePriority=Speed  RndMeth=Simplest
  speed_hp_filt1 : Subsystem
  torque_for_brake_operation_sign_negative : RelationalOperator  Operator=<  OutDataTypeStr=boolean  RndMeth=Simplest  InputSameDT=off
  pos_control_active_flag_VA : Outport
  position_control_trq_output_VA : Outport  Port=2
  speed_filt : Outport  Port=3
  wires:
  Constant13/1 -> torque_for_brake_operation_sign_negative/2
  Compare To Constant3/1 -> Logical Operator/2
  brake_torque_total/1 -> Switch8/3, Max/1, torque_for_brake_operation_sign_negative/1, delta_speed_to_torque3/2
  pos_ctrl_blending/1(Out1) -> position_control_trq_output_VA/1
  Constant17/1 -> delta_n/1
  Abs/1 -> delta_n/2
  Saturation2/1 -> Switch8/1
  pos_ctrl_active/1 -> Logical Operator/1
  Product5/1 -> Product9/2
  Data Type Conversion1/1 -> Product9/1
  torque_for_brake_operation_sign_negative/1 -> Logical Operator1/2
  Product9/1 -> Max/2
  Max/1 -> Saturation2/1
  Logical Operator1/1 -> Switch8/2
  delta_speed_to_torque/1 -> VariabGainOut_VA/3
  Switch8/1 -> pos_ctrl_blending/1(In1)  "position_control_trq_output"
  Logical Operator/1 -> Logical Operator1/1, pos_control_active_flag_VA/1, Data Type Conversion1/1
  Compare To Constant4/1 -> Logical Operator/3
  speed_dep_pt1/1 -> pos_ctrl_blending/2(In2)
  speed_act_VA/1 -> speed_hp_filt1/1(speed_act)
  speed_hp_filt1/1(H2_result) -> speed_filt/1, Compare To Constant3/1, speed_dep_pt1/1, Compare To Constant4/1, Abs/1  "SPEED_FILT_H2"
  delta_speed_to_torque3/1 -> VariabGainOut_VA/1
  activate_var_gain_VA/1 -> VariabGainOut_VA/2
  delta_n/1 -> delta_speed_to_torque3/1, Product5/2, delta_speed_to_torque/1
  VariabGainOut_VA/1 -> Product5/1

== system SoftStop_Standalone/SoftStop/State_Standstill_HA/speed_hp_filt ==
  speed_act : Inport
  2-D Lookup Table1 : Lookup_n-D  NumberOfTableDimensions=1  BreakpointsForDimension1=iStop_Standstill_Axis_SpeedAct_HA  BreakpointsForDimension2=[1:3]  Table=iStop_Standstill_Hp_Filt_HA  ExtrapMethod=Clip  UseLastTableValue=on  InternalRulePriority=Speed  RndMeth=Simplest
  Add1 : Sum  Inputs=+-
  Subsystem : Subsystem  AncestorBlock=AntiJerk_rear/AntiJerk_rear/State_Standstill_VA/speed_hp_filt/Subsystem
  Subsystem1 : Subsystem  AncestorBlock=AntiJerk_rear/AntiJerk_rear/State_Standstill_VA/speed_hp_filt/Subsystem1
  H2_result : Outport
  wires:
  Subsystem1/1(Out1) -> Add1/2
  Subsystem/1(Out1) -> Subsystem1/1(HP1_in)
  Add1/1 -> H2_result/1
  speed_act/1 -> 2-D Lookup Table1/1, Add1/1, Subsystem/1(HP1_in)  "HP1_in"
  2-D Lookup Table1/1 -> Subsystem1/2(Input), Subsystem/2(In2)

== system SoftStop_Standalone/SoftStop/State_Standstill_VA/speed_hp_filt ==
  speed_act : Inport
  2-D Lookup Table1 : Lookup_n-D  NumberOfTableDimensions=1  BreakpointsForDimension1=iStop_Standstill_Axis_SpeedAct_VA  BreakpointsForDimension2=[1:3]  Table=iStop_Standstill_Hp_Filt_VA  ExtrapMethod=Clip  UseLastTableValue=on  InternalRulePriority=Speed  RndMeth=Simplest
  Add1 : Sum  Inputs=+-
  Subsystem : Subsystem  AncestorBlock=AntiJerk_rear/AntiJerk_rear/State_Standstill_VA/speed_hp_filt/Subsystem
  Subsystem1 : Subsystem  AncestorBlock=AntiJerk_rear/AntiJerk_rear/State_Standstill_VA/speed_hp_filt/Subsystem1
  H2_result : Outport
  wires:
  2-D Lookup Table1/1 -> Subsystem1/2(Input), Subsystem/2(In2)
  Add1/1 -> H2_result/1
  speed_act/1 -> 2-D Lookup Table1/1, Add1/1, Subsystem/1(HP1_in)  "HP1_in"
  Subsystem/1(Out1) -> Subsystem1/1(HP1_in)
  Subsystem1/1(Out1) -> Add1/2

== system SoftStop_Standalone/SoftStop/pos_ctrl_HA/pos_ctrl_blending ==
  In1 : Inport
  In2 : Inport  Port=2
  Add1 : Sum
  Add2 : Sum  Inputs=+-
  Product10 : Product
  Unit Delay : UnitDelay  SampleTime=-1  HasFrameUpgradeWarning=on
  Out1 : Outport
  wires:
  In1/1 -> Add2/1
  Add1/1 -> Unit Delay/1, Out1/1
  In2/1 -> Product10/2
  Add2/1 -> Product10/1
  Product10/1 -> Add1/2
  Unit Delay/1 -> Add2/2, Add1/1

== system SoftStop_Standalone/SoftStop/pos_ctrl_HA/speed_hp_filt1 ==
  speed_act : Inport
  2-D Lookup Table1 : Lookup_n-D  NumberOfTableDimensions=1  BreakpointsForDimension1=iStop_PosCtrl_Axis_SpeedActRear  BreakpointsForDimension2=[1:3]  Table=iStop_PosCtrl_Hp_Filt_HA  ExtrapMethod=Clip  UseLastTableValue=on  InternalRulePriority=Speed  RndMeth=Simplest
  Add2 : Sum  Inputs=+-
  Subsystem2 : Subsystem
  Subsystem3 : Subsystem
  H2_result : Outport
  wires:
  speed_act/1 -> Subsystem2/1(HP1_in), Add2/1, 2-D Lookup Table1/1
  Add2/1 -> H2_result/1
  Subsystem2/1(Out1) -> Subsystem3/1(HP1_in)
  Subsystem3/1(Out1) -> Add2/2
  2-D Lookup Table1/1 -> Subsystem2/2(In2), Subsystem3/2(Input)

== system SoftStop_Standalone/SoftStop/pos_ctrl_VA/pos_ctrl_blending ==
  In1 : Inport
  In2 : Inport  Port=2
  Add1 : Sum
  Add2 : Sum  Inputs=+-
  Product10 : Product
  Unit Delay : UnitDelay  SampleTime=-1  HasFrameUpgradeWarning=on
  Out1 : Outport
  wires:
  Unit Delay/1 -> Add1/1, Add2/2
  Product10/1 -> Add1/2
  Add2/1 -> Product10/1
  In2/1 -> Product10/2
  Add1/1 -> Out1/1, Unit Delay/1
  In1/1 -> Add2/1

== system SoftStop_Standalone/SoftStop/pos_ctrl_VA/speed_hp_filt1 ==
  speed_act : Inport
  2-D Lookup Table1 : Lookup_n-D  NumberOfTableDimensions=1  BreakpointsForDimension1=iStop_PosCtrl_Axis_SpeedAct_VA  BreakpointsForDimension2=[1:3]  Table=iStop_PosCtrl_Hp_Filt_VA  ExtrapMethod=Clip  UseLastTableValue=on  InternalRulePriority=Speed  RndMeth=Simplest
  Add2 : Sum  Inputs=+-
  Subsystem2 : Subsystem
  Subsystem3 : Subsystem
  H2_result : Outport
  wires:
  2-D Lookup Table1/1 -> Subsystem3/2(Input), Subsystem2/2(In2)
  Subsystem3/1(Out1) -> Add2/2
  Subsystem2/1(Out1) -> Subsystem3/1(HP1_in)
  Add2/1 -> H2_result/1
  speed_act/1 -> Add2/1, Subsystem2/1(HP1_in), 2-D Lookup Table1/1  "HP1_in"

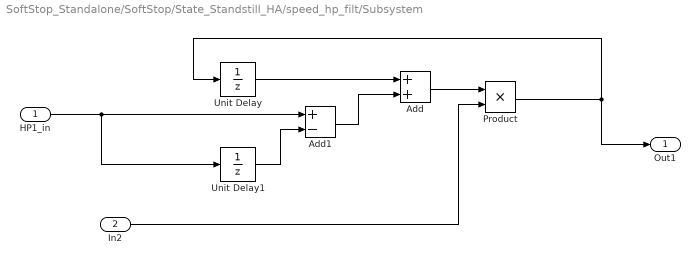
== system SoftStop_Standalone/SoftStop/State_Standstill_HA/speed_hp_filt/Subsystem ==
  HP1_in : Inport
  In2 : Inport  Port=2
  Add : Sum
  Add1 : Sum  Inputs=+-
  Product : Product
  Unit Delay : UnitDelay  SampleTime=-1  HasFrameUpgradeWarning=on
  Unit Delay1 : UnitDelay  SampleTime=-1  HasFrameUpgradeWarning=on
  Out1 : Outport
  wires:
  Add/1 -> Product/1
  HP1_in/1 -> Unit Delay1/1, Add1/1
  Unit Delay1/1 -> Add1/2
  Product/1 -> Out1/1, Unit Delay/1
  In2/1 -> Product/2
  Unit Delay/1 -> Add/1
  Add1/1 -> Add/2

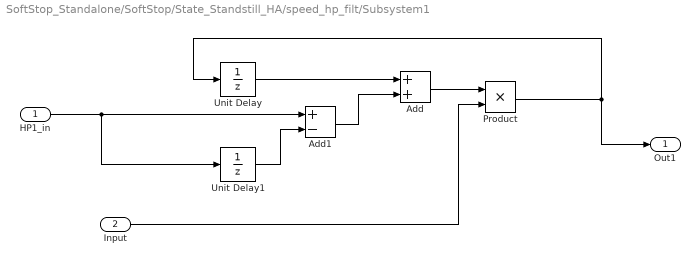
== system SoftStop_Standalone/SoftStop/State_Standstill_HA/speed_hp_filt/Subsystem1 ==
  HP1_in : Inport
  Input : Inport  Port=2
  Add : Sum
  Add1 : Sum  Inputs=+-
  Product : Product
  Unit Delay : UnitDelay  SampleTime=-1  HasFrameUpgradeWarning=on
  Unit Delay1 : UnitDelay  SampleTime=-1  HasFrameUpgradeWarning=on
  Out1 : Outport
  wires:
  Add/1 -> Product/1
  HP1_in/1 -> Unit Delay1/1, Add1/1
  Unit Delay1/1 -> Add1/2
  Product/1 -> Out1/1, Unit Delay/1
  Input/1 -> Product/2
  Unit Delay/1 -> Add/1
  Add1/1 -> Add/2

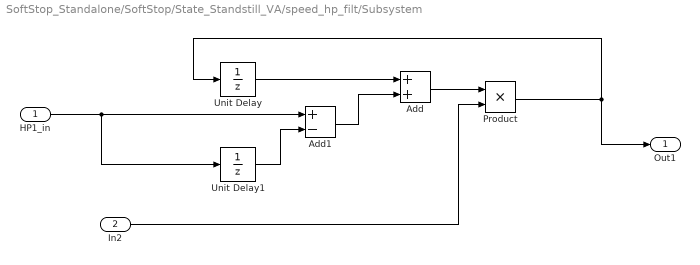
== system SoftStop_Standalone/SoftStop/State_Standstill_VA/speed_hp_filt/Subsystem ==
  HP1_in : Inport
  In2 : Inport  Port=2
  Add : Sum
  Add1 : Sum  Inputs=+-
  Product : Product
  Unit Delay : UnitDelay  SampleTime=-1  HasFrameUpgradeWarning=on
  Unit Delay1 : UnitDelay  SampleTime=-1  HasFrameUpgradeWarning=on
  Out1 : Outport
  wires:
  Add/1 -> Product/1
  HP1_in/1 -> Unit Delay1/1, Add1/1
  Unit Delay1/1 -> Add1/2
  Product/1 -> Out1/1, Unit Delay/1
  In2/1 -> Product/2
  Unit Delay/1 -> Add/1
  Add1/1 -> Add/2

== system SoftStop_Standalone/SoftStop/State_Standstill_VA/speed_hp_filt/Subsystem1 ==
  HP1_in : Inport
  Input : Inport  Port=2
  Add : Sum
  Add1 : Sum  Inputs=+-
  Product : Product
  Unit Delay : UnitDelay  SampleTime=-1  HasFrameUpgradeWarning=on
  Unit Delay1 : UnitDelay  SampleTime=-1  HasFrameUpgradeWarning=on
  Out1 : Outport
  wires:
  Add/1 -> Product/1
  HP1_in/1 -> Unit Delay1/1, Add1/1
  Unit Delay1/1 -> Add1/2
  Product/1 -> Out1/1, Unit Delay/1
  Input/1 -> Product/2
  Unit Delay/1 -> Add/1
  Add1/1 -> Add/2

== system SoftStop_Standalone/SoftStop/pos_ctrl_HA/speed_hp_filt1/Subsystem2 ==
  HP1_in : Inport
  In2 : Inport  Port=2
  Add : Sum
  Add1 : Sum  Inputs=+-
  Product : Product  OutDataTypeStr=double
  Unit Delay : UnitDelay  SampleTime=-1  HasFrameUpgradeWarning=on
  Unit Delay1 : UnitDelay  SampleTime=-1  HasFrameUpgradeWarning=on
  Out1 : Outport
  wires:
  Add1/1 -> Add/2
  Unit Delay/1 -> Add/1
  In2/1 -> Product/2
  Product/1 -> Unit Delay/1, Out1/1
  Unit Delay1/1 -> Add1/2
  HP1_in/1 -> Add1/1, Unit Delay1/1
  Add/1 -> Product/1

== system SoftStop_Standalone/SoftStop/pos_ctrl_HA/speed_hp_filt1/Subsystem3 ==
  HP1_in : Inport
  Input : Inport  Port=2
  Add : Sum
  Add1 : Sum  Inputs=+-
  Product : Product
  Unit Delay : UnitDelay  SampleTime=-1  HasFrameUpgradeWarning=on
  Unit Delay1 : UnitDelay  SampleTime=-1  HasFrameUpgradeWarning=on
  Out1 : Outport
  wires:
  Add1/1 -> Add/2
  Unit Delay/1 -> Add/1
  Input/1 -> Product/2
  Product/1 -> Unit Delay/1, Out1/1
  Unit Delay1/1 -> Add1/2
  HP1_in/1 -> Add1/1, Unit Delay1/1
  Add/1 -> Product/1

== system SoftStop_Standalone/SoftStop/pos_ctrl_VA/speed_hp_filt1/Subsystem2 ==
  HP1_in : Inport
  In2 : Inport  Port=2
  Add : Sum
  Add1 : Sum  Inputs=+-
  Product : Product  OutDataTypeStr=double
  Unit Delay : UnitDelay  SampleTime=-1  HasFrameUpgradeWarning=on
  Unit Delay1 : UnitDelay  SampleTime=-1  HasFrameUpgradeWarning=on
  Out1 : Outport
  wires:
  Add/1 -> Product/1
  HP1_in/1 -> Unit Delay1/1, Add1/1
  Unit Delay1/1 -> Add1/2
  Product/1 -> Out1/1, Unit Delay/1
  In2/1 -> Product/2
  Unit Delay/1 -> Add/1
  Add1/1 -> Add/2

== system SoftStop_Standalone/SoftStop/pos_ctrl_VA/speed_hp_filt1/Subsystem3 ==
  HP1_in : Inport
  Input : Inport  Port=2
  Add : Sum
  Add1 : Sum  Inputs=+-
  Product : Product
  Unit Delay : UnitDelay  SampleTime=-1  HasFrameUpgradeWarning=on
  Unit Delay1 : UnitDelay  SampleTime=-1  HasFrameUpgradeWarning=on
  Out1 : Outport
  wires:
  Add/1 -> Product/1
  HP1_in/1 -> Unit Delay1/1, Add1/1
  Unit Delay1/1 -> Add1/2
  Product/1 -> Out1/1, Unit Delay/1
  Input/1 -> Product/2
  Unit Delay/1 -> Add/1
  Add1/1 -> Add/2
